simulink model "ISReferenceApplication"  (R2024b)
settings: Solver=ode4  StartTime=0.0  StopTime=60  FixedStep=1e-3  RelTol=5e-2
model workspace (MAT data in the model file):
  Downshift_Speeds = [9.5625 12.9375 16.3125 19.6875 23.0625 26.4375 29.8125 33.1875 36.5625 39.9375 43.3125 46.6875 ... (28 elements, 4x7)]
  EngRevLim = 7000
  Pedal_Positions = [0.1 0.4 0.5 0.9]
  Upshift_Speeds = [12.9375 16.3125 19.6875 33 26.4375 29.8125 33.1875 52.5 39.9375 43.3125 46.6875 77.25 ... (28 elements, 4x7)]
  VEH : object (value not decoded)
  rayDirections = [0 0 0 0 0 0 0 0 0 0 0 0 ... (363 elements, 121x3)]
  rayLengths = [20 20 20 20 20 20 20 20 20 20 20 20 ... (121 elements, 121x1)]
  rayOrigins = [0.5 0.4 0.3 0.2 0.1 0 -0.1 -0.2 -0.3 -0.4 -0.5 0.5 ... (363 elements, 121x3)]
  temp : object (value not decoded)
symbols that are objects in the model workspace (value not decoded): temp, VEH
undefined symbols (not defined in the file): DiscIntNeverNeededParam, Sim3dSensor
libraries: simulink x14, autolibutils x7, slpidlib x2, vehdynlibviscommon x2, sim3dgroundtruthsensorlib x2, autolibtranscontrolscommon x1, autolibshared x1, vehdynlibdriver x1, sharedtransform x1, vehdynlibsens x1, vehdynlibscenariocommon x1, sim3dlib x1
(part 3 of 4)

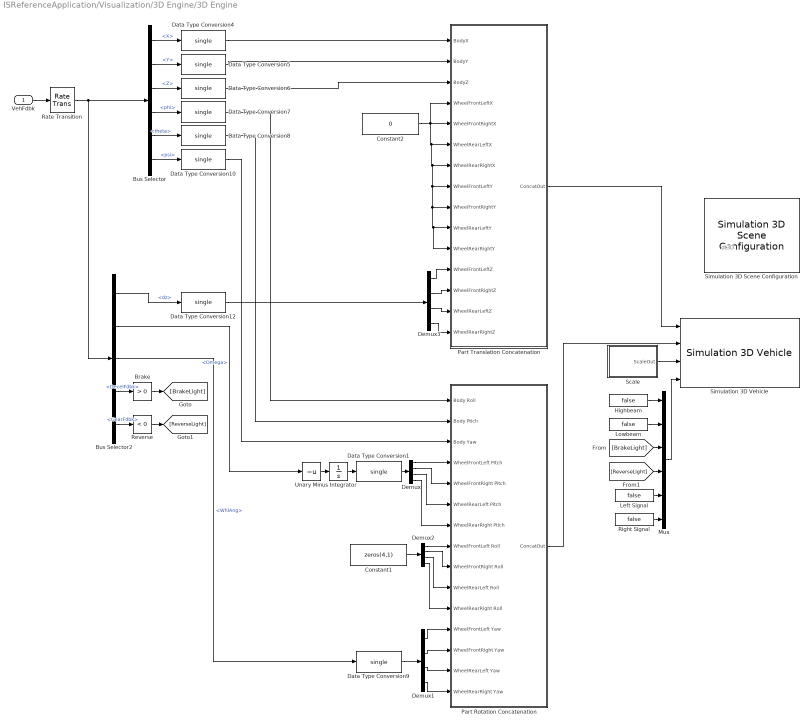
== system ISReferenceApplication/Visualization/3D Engine/3D Engine ==
  note: dt3D
  VehFdbk : Inport
  Brake : simulink/Logic and Bit Operations/Compare To Constant  relop=>  const=0  OutDataTypeStr=boolean  ZeroCross=off
  Bus Selector : BusSelector  OutputSignals=Body.InertFrm.Geom.Disp.X,Body.InertFrm.Geom.Disp.Y,Body.InertFrm.Geom.Disp.Z,Body.InertFrm.Cg.Ang.phi,Body.InertFrm.Cg.Ang.theta,Body.InertFrm.Cg.Ang.psi
  Bus Selector2 : BusSelector  OutputSignals=Wheels.TireFrame.dz,Wheels.TireFrame.Omega,Driveline.WhlAng,Driver.DecelFdbk,Driver.GearFdbk
  Constant1 : Constant  Value=zeros(4,1)  OutDataTypeStr=single
  Constant2 : Constant  Value=0  OutDataTypeStr=single
  Data Type Conversion{1,4..10,12} (9 alike) : DataTypeConversion  OutDataTypeStr=single  SaturateOnIntegerOverflow=off  RndMeth=Floor
  Demux{,1..3} (4 alike) : Demux
  Highbeam : Constant  Value=false
  Integrator : Integrator  WrapState=on  WrappedStateUpperValue=2*pi  WrappedStateLowerValue=0  ZeroCross=off
  Left Signal : Constant  Value=false
  Lowbeam : Constant  Value=false
  Mux : Mux  Inputs=6
  Part Rotation Concatenation : Subsystem
  Part Translation Concatenation : Subsystem
  Rate Transition : RateTransition  OutPortSampleTime=dt3D
  Reverse : simulink/Logic and Bit Operations/Compare To Constant  relop=<  const=0  OutDataTypeStr=boolean  ZeroCross=off
  Right Signal : Constant  Value=false
  Scale : Subsystem
  Simulation 3D Scene Configuration : sim3dlib/Simulation 3D Scene Configuration  Priority=0  ProjectFormat=Default Scenes  SceneDesc=Open surface  ProjectName=C:\Program Files\MATLAB\R2024b\toolbox\shared\sim3d_projects\automotive_project_windows\UE\WindowsNoEditor\VehicleSimulation.exe  ScenePath=/Game/Maps/HwStrght  EnableOpenDRIVE=off  vehTagList={'Custom';'Scene Origin';'SimulinkVehicle1'}  vehTag=SimulinkVehicle1  FreeCameraInitialTranslation=[0, 0, 0]  FreeCameraDefaultInitialTranslation=[-6, 0, 2]  FreeCameraInitialRotation=[0, 0, 0]  FreeCameraDefaultInitialRotation=[0, -15, 0]  OpVisEn=off  Ts=dt3D  EnableWindow=on  EnableRemoteAccess=off  EnableWeather=off  SunAzimuth=90  SunAltitude=40.0  EnableGeospatialSun=off  Latitude=0  Longitude=0  Date=2023-01-01  Time=10:30:00  GeoTimeZone=-5.0  SunDaylightSaving=off  wind=1  clouds=10  EnableVolumetricClouds=off  CloudCoverage=0  CloudAltitude=6  fog=0  rain=0  RaindropsEffect=off  SnowDensity=0  EnableGeospatial=off  UseTrueOrigin=off  OriginHeight=200  OriginLatitude=40.744652  OriginLongitude=-73.988864  MapStyle=Aerial  AdditionalAssetIDs=[]  UseAdvancedSunSky=off  SolarTime=11  TimeZone=-5  Day=21  Month=9  Year=2022  UseDaylightSavingTime=on  DSTStartDay=10  DSTStartMonth=3  DSTEndDay=3  DSTEndMonth=11  DSTSwitchHour=2  sensorTag=MainCamera1  sensorId=1  sensorName=MainCamera1  mountLoc=Origin  offsetFlag=off  tmountOffset=[0, 0, 0]  rmountOffset=[0, 0, 0]  HorizontalResolution=1280  VerticalResolution=720  HorizontalFOV=60  mountPoint=[0 0 0]  mountOrientation=[0 0 0]  aMode=2  ID=1  GeoTrigger=Inactive
      settings: LibrarySourceBlock=vdynlib/Vehicle Scenarios/Sim3D/Sim3D Core/Simulation 3D Scene Configuration
  Simulation 3D Vehicle : sim3dautolib/Simulation 3D Vehicle  Priority=-1  PassVehMesh=Sport utility vehicle  MeshPath=/MathWorksSimulation/Vehicles/Muscle/Meshes/SK_MuscleCar.SK_MuscleCar  VehColor=Red  ActorName=SimulinkVehicle1  VehLightsControl=on  HeadlightColor=[ 1, 1, 1 ]  HighBeamIntensity=100000  LowBeamIntensity=60000  HighBeamConeAngle=1.22  LowBeamConeAngle=1.22  LeftHeadlightOrientation=[ 0, 0 ]  RightHeadlightOrientation=[ 0, 0 ]  BrakelightIntensity=500  ReverselightIntensity=500  SignallightIntensity=500  SignallightPeriod=1  SignalPulseWidth=50  Translation=[VEH.InitialLongPosition VEH.InitialLatPosition -VEH.InitialVertPosition; 0 0 0; 0 0 0; 0 0 0; 0 0 0]  Rotation=[VEH.InitialRollAngle VEH.InitialPitchAngle VEH.InitialYawAngle; 0 0 0; 0 0 0; 0 0 0; 0 0 0]  Scale=ones( 5, 3 )  SampleTime=dt3D  ActorType=SimulinkVehicle  ID=1  aMode=2  ActorTag=SimulinkVehicle1
  Unary Minus : UnaryMinus
  wires:
  Unary Minus/1 -> Integrator/1
  Bus Selector2/1 -> Data Type Conversion12/1  "<dz>"
  Rate Transition/1 -> Bus Selector/1, Bus Selector2/1
  Scale/1(ScaleOut) -> Simulation 3D Vehicle/3
  Demux/4 -> Part Rotation Concatenation/7(WheelRearRight Ptich)
  Demux/3 -> Part Rotation Concatenation/6(WheelRearLeft Pitch)
  Demux/2 -> Part Rotation Concatenation/5(WheelFrontRight Pitch)
  Demux/1 -> Part Rotation Concatenation/4(WheelFrontLeft Pitch)
  Constant1/1 -> Demux2/1
  Bus Selector/4 -> Data Type Conversion7/1  "<phi>"
  Part Rotation Concatenation/1(ConcatOut) -> Simulation 3D Vehicle/2
  Part Translation Concatenation/1(ConcatOut) -> Simulation 3D Vehicle/1
  Data Type Conversion12/1 -> Demux3/1
  Demux3/4 -> Part Translation Concatenation/15(WheelRearRightZ)
  Demux3/3 -> Part Translation Concatenation/14(WheelRearLeftZ)
  Demux3/1 -> Part Translation Concatenation/12(WheelFrontLeftZ)
  Demux3/2 -> Part Translation Concatenation/13(WheelFrontRightZ)
  VehFdbk/1 -> Rate Transition/1
  Data Type Conversion6/1 -> Part Translation Concatenation/3(BodyZ)
  Demux1/4 -> Part Rotation Concatenation/15(WheelRearRight Yaw)
  Demux1/3 -> Part Rotation Concatenation/14(WheelRearLeft Yaw)
  Demux2/1 -> Part Rotation Concatenation/8(WheelFrontLeft Roll)
  Demux2/2 -> Part Rotation Concatenation/9(WheelFrontRight Roll)
  Demux2/3 -> Part Rotation Concatenation/10(WheelRearLeft Roll)
  Demux2/4 -> Part Rotation Concatenation/11(WheelRearRight Roll)
  Bus Selector2/3 -> Data Type Conversion9/1  "<WhlAng>"
  Bus Selector2/2 -> Unary Minus/1  "<Omega>"
  Data Type Conversion9/1 -> Demux1/1
  Demux1/1 -> Part Rotation Concatenation/12(WheelFrontLeft Yaw)
  Demux1/2 -> Part Rotation Concatenation/13(WheelFrontRight Yaw)
  Integrator/1 -> Data Type Conversion1/1
  Data Type Conversion1/1 -> Demux/1
  Data Type Conversion8/1 -> Part Rotation Concatenation/2(Body Ptich)
  Data Type Conversion5/1 -> Part Translation Concatenation/2(BodyY)
  Data Type Conversion10/1 -> Part Rotation Concatenation/3(Body Yaw)
  Constant2/1 -> Part Translation Concatenation/5(WheelFrontRightX), Part Translation Concatenation/6(WheelRearLeftX), Part Translation Concatenation/7(WheelRearRightX), Part Translation Concatenation/8(WheelFrontLeftY), Part Translation Concatenation/9(WheelFrontRightY), Part Translation Concatenation/10(WheelRearLeftY), Part Translation Concatenation/11(WheelRearRightY), Part Translation Concatenation/4(WheelFrontLeftX)
  Data Type Conversion4/1 -> Part Translation Concatenation/1(BodyX)
  Data Type Conversion7/1 -> Part Rotation Concatenation/1(Body Roll)
  Bus Selector/1 -> Data Type Conversion4/1  "<X>"
  Bus Selector/2 -> Data Type Conversion5/1  "<Y>"
  Bus Selector/3 -> Data Type Conversion6/1  "<Z>"
  Bus Selector/6 -> Data Type Conversion10/1  "<psi>"
  Bus Selector/5 -> Data Type Conversion8/1  "<theta>"
  [BrakeLight] -> Mux/3
  Mux/1 -> Simulation 3D Vehicle/4
  Brake/1 -> [BrakeLight]
  Highbeam/1 -> Mux/1
  Reverse/1 -> [ReverseLight]
  [ReverseLight] -> Mux/4
  Lowbeam/1 -> Mux/2
  Right Signal/1 -> Mux/6
  Left Signal/1 -> Mux/5
  Bus Selector2/4 -> Brake/1  "<DecelFdbk>"
  Bus Selector2/5 -> Reverse/1  "<GearFdbk>"

== system ISReferenceApplication/Visualization/3D Engine/3D Engine Disabled ==
  VehFdbk : Inport
  Terminator : Terminator
  wires:
  VehFdbk/1 -> Terminator/1

== system ISReferenceApplication/Visualization/ISO 15037-1:2006/Disabled ==
  VehFdbk : Inport
  Terminator1 : Terminator
  wires:
  VehFdbk/1 -> Terminator1/1

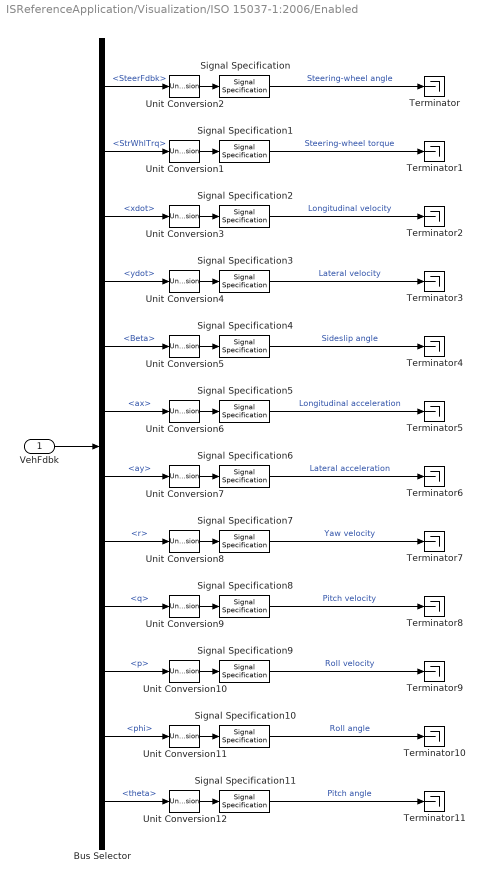
== system ISReferenceApplication/Visualization/ISO 15037-1:2006/Enabled ==
  VehFdbk : Inport
  Bus Selector : BusSelector  OutputSignals=Driver.SteerFdbk,Steering.StrWhlTrq,Body.BdyFrm.Cg.Vel.xdot,Body.BdyFrm.Cg.Vel.ydot,Body.BdyFrm.Cg.Ang.Beta,Body.BdyFrm.Cg.Acc.ax,Body.BdyFrm.Cg.Acc.ay,Body.BdyFrm.Cg.AngVel.r,Body.BdyFrm.Cg.AngVel.q,Body.BdyFrm.Cg.AngVel.p,Body.InertFrm.Cg.Ang.phi,Body.InertFrm.Cg.Ang.theta
  Signal Specification{,4,10..11} (4 alike) : SignalSpecification  Unit=deg
  Signal Specification1 : SignalSpecification  Unit=N*m
  Signal Specification2 : SignalSpecification  Unit=km/h
  Signal Specification3 : SignalSpecification  Unit=m/s
  Signal Specification5 : SignalSpecification  Unit=m/s^2
  Signal Specification6 : SignalSpecification  Unit=m/s^2
  Signal Specification7 : SignalSpecification  Unit=deg/s
  Signal Specification8 : SignalSpecification  Unit=deg/s
  Signal Specification9 : SignalSpecification  Unit=deg/s
  Terminator{,1..11} (12 alike) : Terminator
  Unit Conversion{1..12} (12 alike) : UnitConversion
  wires:
  Bus Selector/12 -> Unit Conversion12/1  "<theta>"
  Signal Specification11/1 -> Terminator11/1  "Pitch angle"
  Unit Conversion12/1 -> Signal Specification11/1
  Bus Selector/11 -> Unit Conversion11/1  "<phi>"
  Unit Conversion11/1 -> Signal Specification10/1
  Signal Specification10/1 -> Terminator10/1  "Roll angle"
  Bus Selector/10 -> Unit Conversion10/1  "<p>"
  Signal Specification9/1 -> Terminator9/1  "Roll velocity"
  Unit Conversion10/1 -> Signal Specification9/1
  Bus Selector/9 -> Unit Conversion9/1  "<q>"
  Unit Conversion9/1 -> Signal Specification8/1
  Signal Specification8/1 -> Terminator8/1  "Pitch velocity"
  Bus Selector/8 -> Unit Conversion8/1  "<r>"
  Signal Specification7/1 -> Terminator7/1  "Yaw velocity"
  Unit Conversion8/1 -> Signal Specification7/1
  Bus Selector/7 -> Unit Conversion7/1  "<ay>"
  Unit Conversion7/1 -> Signal Specification6/1
  Signal Specification6/1 -> Terminator6/1  "Lateral acceleration"
  Bus Selector/6 -> Unit Conversion6/1  "<ax>"
  Signal Specification5/1 -> Terminator5/1  "Longitudinal acceleration"
  Unit Conversion6/1 -> Signal Specification5/1
  Bus Selector/5 -> Unit Conversion5/1  "<Beta>"
  Unit Conversion5/1 -> Signal Specification4/1
  Signal Specification4/1 -> Terminator4/1  "Sideslip angle"
  Bus Selector/4 -> Unit Conversion4/1  "<ydot>"
  Signal Specification3/1 -> Terminator3/1  "Lateral velocity"
  Unit Conversion4/1 -> Signal Specification3/1
  Bus Selector/3 -> Unit Conversion3/1  "<xdot>"
  Unit Conversion3/1 -> Signal Specification2/1
  Signal Specification2/1 -> Terminator2/1  "Longitudinal velocity"
  Signal Specification1/1 -> Terminator1/1  "Steering-wheel torque"
  Unit Conversion1/1 -> Signal Specification1/1
  Bus Selector/2 -> Unit Conversion1/1  "<StrWhlTrq>"
  Signal Specification/1 -> Terminator/1  "Steering-wheel angle"
  Unit Conversion2/1 -> Signal Specification/1
  VehFdbk/1 -> Bus Selector/1
  Bus Selector/1 -> Unit Conversion2/1  "<SteerFdbk>"

== system ISReferenceApplication/Controllers/Brake Pressure Control/Bang Bang ABS/Bang-bang controller ==
  in_1 : Inport
  Constant : Constant  Value=0
  Data Type Conversion1 : DataTypeConversion  OutDataTypeStr=double
  Data Type Conversion2 : DataTypeConversion  OutDataTypeStr=double
  Relational Operator : RelationalOperator  Operator=>  OutDataTypeStr=boolean
  Relational Operator1 : RelationalOperator  Operator=<  OutDataTypeStr=boolean
  Sum : Sum  Inputs=+-  InputSameDT=on  SaturateOnIntegerOverflow=on  OutDataTypeStr=Inherit: Same as first input
  out_1 : Outport  InitialOutput=0  VectorParamsAs1DForOutWhenUnconnected=off
  wires:
  Data Type Conversion2/1 -> Sum/2
  Data Type Conversion1/1 -> Sum/1
  Sum/1 -> out_1/1
  Relational Operator/1 -> Data Type Conversion1/1
  Relational Operator1/1 -> Data Type Conversion2/1
  Constant/1 -> Relational Operator/2, Relational Operator1/2
  in_1/1 -> Relational Operator1/1, Relational Operator/1

== system ISReferenceApplication/Controllers/Brake Pressure Control/Bang Bang ABS/Kappa ==
  xdot : Inport
  Omega : Inport  Port=2  Partition=on  PartitionDimension=1  PartitionWidth=1  PartitionOffset=0
  For Each : ForEach  DisableCoverage=on
  MATLAB Function : MATLAB Function  TreatAsAtomicUnit=on
  KappaEst : Outport  ConcatenationDimension=1
  wires:
  MATLAB Function/1(KappaEst) -> KappaEst/1
  xdot/1 -> MATLAB Function/2(xdot)
  Omega/1 -> MATLAB Function/1(Omega)

== system ISReferenceApplication/Controllers/Brake Pressure Control/Five-State ABS and TCS/ABSCtrlForEach ==
  Pref : Inport
  WhlAccel : Inport  Port=2
  WhlSlip : Inport  Port=3
  VehSpd : Inport  Port=4
  Constant7 : Constant  Value=WhlAccelOpt
  Constant8 : Constant  Value=KappaOpt
  For Each Subsystem : Subsystem  TreatAsAtomicUnit=on
  Gain : Gain  Gain=Re
  Saturation1 : Saturate  UpperLimit=1  LowerLimit=-1
  Selector : Selector  InputPortWidth=1  IndexOptions=Index vector (dialog)  Indices=[1 1 1 1]  OutputSizes=1
  Sum : Sum  Inputs=|+-
  Sum1 : Sum  Inputs=|+-
  BrkCtrl : Outport
  BrkFlag : Outport  Port=2
  wires:
  Gain/1 -> Sum/1
  Constant8/1 -> Sum1/2
  WhlSlip/1 -> Saturation1/1
  Constant7/1 -> Sum/2
  Sum1/1 -> For Each Subsystem/1(e1)
  WhlAccel/1 -> Gain/1
  Saturation1/1 -> Sum1/1
  For Each Subsystem/2(Flag) -> BrkFlag/1
  Pref/1 -> Selector/1
  VehSpd/1 -> For Each Subsystem/4(VehSpd)
  For Each Subsystem/1(Pb) -> BrkCtrl/1  "BrkPrsCmdCtrl"
  Selector/1 -> For Each Subsystem/3(Pref)
  Sum/1 -> For Each Subsystem/2(e2)

== system ISReferenceApplication/Controllers/Brake Pressure Control/Five-State ABS and TCS/TCSCtrlForEach ==
  WhlAccel : Inport
  WhlSlip : Inport  Port=2
  AccelFdbk : Inport  Port=3
  PbFdbk : Inport  Port=4
  Constant7 : Constant  Value=WhlAccelOpt
  Constant8 : Constant  Value=KappaOpt
  For Each Subsystem : Subsystem  TreatAsAtomicUnit=on
  Gain : Gain  Gain=Re
  Interpreted MATLAB Function : MATLABFcn  MATLABFcn=abs((u(1)+u(2)) - (u(3) + u(4)))/2
  Saturation1 : Saturate  UpperLimit=1  LowerLimit=-1
  Selector : Selector  InputPortWidth=1  IndexOptions=Index vector (dialog)  Indices=[1 1 1 1]  OutputSizes=1
  Sum : Sum  Inputs=|+-
  Sum1 : Sum  Inputs=|+-
  BrkCtrl : Outport
  BrkFlag : Outport  Port=2
  wires:
  Gain/1 -> Sum/1
  Constant8/1 -> Sum1/2
  WhlSlip/1 -> Saturation1/1
  Constant7/1 -> Sum/2
  Sum1/1 -> For Each Subsystem/1(e1)
  WhlAccel/1 -> Gain/1
  Saturation1/1 -> Interpreted MATLAB Function/1, Sum1/1
  For Each Subsystem/2(Flag) -> BrkFlag/1
  AccelFdbk/1 -> Selector/1
  For Each Subsystem/1(Pb) -> BrkCtrl/1  "BrkPrsCmdCtrl"
  Selector/1 -> For Each Subsystem/4(AccelFdbk)
  Sum/1 -> For Each Subsystem/3(e2)
  Interpreted MATLAB Function/1 -> For Each Subsystem/2(Enb)
  PbFdbk/1 -> For Each Subsystem/5(PbFdbk)

== system ISReferenceApplication/Controllers/Brake Pressure Control/Five-State ABS and TCS/Wheel Accel and Slip Estimator ==
  Omega : Inport
  Accel : Inport  Port=2
  Demux : Demux  Outputs=3
  Discrete-Time Integrator : DiscreteIntegrator  IntegratorMethod=Integration: Trapezoidal  SampleTime=-1  ICPrevOutput=DiscIntNeverNeededParam  ICPrevScaledInput=DiscIntNeverNeededParam
  Kappa : Subsystem  TreatAsAtomicUnit=on
  Terminator : Terminator
  Terminator1 : Terminator
  Wheel Accel : Subsystem  TreatAsAtomicUnit=on
  <WhlAccel> : Outport
  <Kappa> : Outport  Port=2
  <xdot> : Outport  Port=3
  wires:
  Accel/1 -> Demux/1
  Discrete-Time Integrator/1 -> <xdot>/1, Kappa/1(xdot)
  Demux/1 -> Discrete-Time Integrator/1
  Demux/2 -> Terminator/1
  Demux/3 -> Terminator1/1
  Omega/1 -> Kappa/2(Omega), Wheel Accel/1(Omega)
  Wheel Accel/1(WhlAccel) -> <WhlAccel>/1
  Kappa/1(KappaEst) -> <Kappa>/1

== system ISReferenceApplication/Controllers/ECU/Torque Cmd/Rev Limiter Control ==
  TrqCmd : Inport
  EngSpd : Inport  Port=2
  1-D Lookup Table : Lookup_n-D  NumberOfTableDimensions=1  BreakpointsForDimension1=[1 1.01]  Table=[1 0]  ExtrapMethod=Clip  InternalRulePriority=Speed  RndMeth=Simplest
  Constant : Constant  Value=EngRevLim
  Product : Product
  Product1 : Product  Inputs=*/
  TrqCmdRevLimited : Outport  VectorParamsAs1DForOutWhenUnconnected=off
  wires:
  EngSpd/1 -> Product1/1
  Product/1 -> TrqCmdRevLimited/1
  1-D Lookup Table/1 -> Product/2
  TrqCmd/1 -> Product/1
  Constant/1 -> Product1/2
  Product1/1 -> 1-D Lookup Table/1

== system ISReferenceApplication/Controllers/Transmission Controller/Transmission Controller/TCM ==
  AccCmd : Inport
  EngSpd : Inport  Port=2
  Omega : Inport  Port=3  Unit=rad/s
  function : TriggerPort  TriggerType=function-call  VariantControl=Variant
  Gain : Gain  Gain=.3065/4
  Neutral Select : Subsystem
  Signal Specification1 : SignalSpecification  Unit=m/s
  Signal Specification2 : SignalSpecification  Unit=km/hr
  Speed LPF : DiscreteTransferFcn  Numerator=[0.000000000000000 0.009950166250832 ]  Denominator=[1.000000000000000 -0.990049833749168 ]  mask(DiscretizedDiscreteTransferFcn){}
      mask init:
      | %zoh
  Sum of Elements : Sum  Inputs=+
  TCM Shift Controller : Stateflow chart  TreatAsAtomicUnit=on
  Unit Conversion1 : UnitConversion
  GearCmd : Outport  VectorParamsAs1DForOutWhenUnconnected=off
  wires:
  Signal Specification2/1 -> Speed LPF/1
  TCM Shift Controller/1(GearCmd) -> GearCmd/1  "GearCmd"
  AccCmd/1 -> Neutral Select/1(AccCmd), TCM Shift Controller/2(pedal)  "AccCmd"
  Neutral Select/1(Neutral Select) -> TCM Shift Controller/3(Neutral)
  EngSpd/1 -> Neutral Select/2(EngSpd)
  Speed LPF/1 -> TCM Shift Controller/1(speed)
  Unit Conversion1/1 -> Signal Specification2/1
  Omega/1 -> Sum of Elements/1
  Gain/1 -> Signal Specification1/1
  Signal Specification1/1 -> Unit Conversion1/1
  Sum of Elements/1 -> Gain/1

== system ISReferenceApplication/Environment/Ground Feedback/3D Engine/3D Engine Source ==
  VehFdbk : Inport
  Multiple Points : Subsystem  VariantControl=terrType==2
  Single Point : Subsystem  VariantControl=terrType ==1
  z : Outport
  DCM : Outport  Port=2

== system ISReferenceApplication/Visualization/3D Engine/3D Engine/Part Rotation Concatenation ==
  Body Roll : Inport
  Body Ptich : Inport  Port=2
  Body Yaw : Inport  Port=3
  WheelFrontLeft Pitch : Inport  Port=4
  WheelFrontRight Pitch : Inport  Port=5
  WheelRearLeft Pitch : Inport  Port=6
  WheelRearRight Ptich : Inport  Port=7
  WheelFrontLeft Roll : Inport  Port=8
  WheelFrontRight Roll : Inport  Port=9
  WheelRearLeft Roll : Inport  Port=10
  WheelRearRight Roll : Inport  Port=11
  WheelFrontLeft Yaw : Inport  Port=12
  WheelFrontRight Yaw : Inport  Port=13
  WheelRearLeft Yaw : Inport  Port=14
  WheelRearRight Yaw : Inport  Port=15
  AllParts : Concatenate  NumInputs=5  Mode=Multidimensional array
  Body : Concatenate  NumInputs=3  Mode=Multidimensional array  ConcatenateDimension=2
  WheelFrontLeft : Concatenate  NumInputs=3  Mode=Multidimensional array  ConcatenateDimension=2
  WheelFrontRight : Concatenate  NumInputs=3  Mode=Multidimensional array  ConcatenateDimension=2
  WheelRearLeft : Concatenate  NumInputs=3  Mode=Multidimensional array  ConcatenateDimension=2
  WheelRearRight : Concatenate  NumInputs=3  Mode=Multidimensional array  ConcatenateDimension=2
  ConcatOut : Outport  VectorParamsAs1DForOutWhenUnconnected=off
  wires:
  Body Yaw/1 -> Body/3
  WheelFrontLeft Yaw/1 -> WheelFrontLeft/3
  WheelFrontLeft/1 -> AllParts/2
  Body/1 -> AllParts/1
  WheelRearLeft/1 -> AllParts/4
  WheelFrontRight/1 -> AllParts/3
  WheelRearRight Yaw/1 -> WheelRearRight/3
  WheelRearLeft Yaw/1 -> WheelRearLeft/3
  AllParts/1 -> ConcatOut/1
  WheelRearRight/1 -> AllParts/5
  WheelFrontRight Yaw/1 -> WheelFrontRight/3
  Body Roll/1 -> Body/1
  Body Ptich/1 -> Body/2
  WheelFrontLeft Pitch/1 -> WheelFrontLeft/2
  WheelFrontLeft Roll/1 -> WheelFrontLeft/1
  WheelFrontRight Roll/1 -> WheelFrontRight/1
  WheelFrontRight Pitch/1 -> WheelFrontRight/2
  WheelRearLeft Roll/1 -> WheelRearLeft/1
  WheelRearLeft Pitch/1 -> WheelRearLeft/2
  WheelRearRight Roll/1 -> WheelRearRight/1
  WheelRearRight Ptich/1 -> WheelRearRight/2

== system ISReferenceApplication/Visualization/3D Engine/3D Engine/Part Translation Concatenation ==
  BodyX : Inport
  BodyY : Inport  Port=2
  BodyZ : Inport  Port=3
  WheelFrontLeftX : Inport  Port=4
  WheelFrontRightX : Inport  Port=5
  WheelRearLeftX : Inport  Port=6
  WheelRearRightX : Inport  Port=7
  WheelFrontLeftY : Inport  Port=8
  WheelFrontRightY : Inport  Port=9
  WheelRearLeftY : Inport  Port=10
  WheelRearRightY : Inport  Port=11
  WheelFrontLeftZ : Inport  Port=12
  WheelFrontRightZ : Inport  Port=13
  WheelRearLeftZ : Inport  Port=14
  WheelRearRightZ : Inport  Port=15
  AllParts : Concatenate  NumInputs=5  Mode=Multidimensional array
  Body : Concatenate  NumInputs=3  Mode=Multidimensional array  ConcatenateDimension=2
  WheelFrontLeft : Concatenate  NumInputs=3  Mode=Multidimensional array  ConcatenateDimension=2
  WheelFrontRight : Concatenate  NumInputs=3  Mode=Multidimensional array  ConcatenateDimension=2
  WheelRearLeft : Concatenate  NumInputs=3  Mode=Multidimensional array  ConcatenateDimension=2
  WheelRearRight : Concatenate  NumInputs=3  Mode=Multidimensional array  ConcatenateDimension=2
  ConcatOut : Outport  VectorParamsAs1DForOutWhenUnconnected=off
  wires:
  BodyX/1 -> Body/1
  BodyZ/1 -> Body/3
  WheelFrontLeftX/1 -> WheelFrontLeft/1
  WheelFrontLeftZ/1 -> WheelFrontLeft/3
  WheelFrontLeftY/1 -> WheelFrontLeft/2
  BodyY/1 -> Body/2
  WheelFrontLeft/1 -> AllParts/2
  WheelRearRightX/1 -> WheelRearRight/1
  Body/1 -> AllParts/1
  WheelRearLeft/1 -> AllParts/4
  WheelFrontRight/1 -> AllParts/3
  WheelRearRightZ/1 -> WheelRearRight/3
  WheelFrontRightY/1 -> WheelFrontRight/2
  WheelFrontRightX/1 -> WheelFrontRight/1
  WheelRearRightY/1 -> WheelRearRight/2
  WheelRearLeftZ/1 -> WheelRearLeft/3
  AllParts/1 -> ConcatOut/1
  WheelRearLeftY/1 -> WheelRearLeft/2
  WheelRearRight/1 -> AllParts/5
  WheelRearLeftX/1 -> WheelRearLeft/1
  WheelFrontRightZ/1 -> WheelFrontRight/3

== system ISReferenceApplication/Visualization/3D Engine/3D Engine/Scale ==
  Constant{1..12,17,32..33} (15 alike) : Constant  OutDataTypeStr=single
  PartConcatenation : Subsystem
  ScaleOut : Outport  VectorParamsAs1DForOutWhenUnconnected=off
  wires:
  Constant10/1 -> PartConcatenation/15(WheelRearRightZ)
  Constant9/1 -> PartConcatenation/14(WheelRearRightY)
  Constant11/1 -> PartConcatenation/13(WheelRearRightX)
  Constant7/1 -> PartConcatenation/12(WheelRearLeftZ)
  Constant6/1 -> PartConcatenation/11(WheelRearLeftY)
  Constant8/1 -> PartConcatenation/10(WheelRearLeftX)
  Constant4/1 -> PartConcatenation/9(WheelFrontRightZ)
  Constant3/1 -> PartConcatenation/8(WheelFrontRightY)
  Constant5/1 -> PartConcatenation/7(WheelFrontRightX)
  Constant2/1 -> PartConcatenation/6(WheelFrontLeftZ)
  Constant1/1 -> PartConcatenation/5(WheelFrontLeftY)
  Constant33/1 -> PartConcatenation/4(WheelFrontLeftX)
  Constant32/1 -> PartConcatenation/3(BodyZ)
  Constant17/1 -> PartConcatenation/2(BodyY)
  Constant12/1 -> PartConcatenation/1(BodyX)
  PartConcatenation/1(ConcatOut) -> ScaleOut/1

== system ISReferenceApplication/Controllers/Brake Pressure Control/Five-State ABS and TCS/ABSCtrlForEach/For Each Subsystem ==
  e1 : Inport  Partition=on  PartitionDimension=1  PartitionWidth=1  PartitionOffset=0
  e2 : Inport  Port=2  Partition=on  PartitionDimension=1  PartitionWidth=1  PartitionOffset=0
  Pref : Inport  Port=3  Partition=on  PartitionDimension=1  PartitionWidth=1  PartitionOffset=0
  VehSpd : Inport  Port=4
  ABSForEachWheel : Stateflow chart  InitFcn=[~]=vehdynicon('vehdynblk',gcb);  TreatAsAtomicUnit=on
  For Each : ForEach  DisableCoverage=on
  Saturation2 : Saturate  UpperLimit=1  LowerLimit=0  ZeroCross=off
  Pb : Outport  ConcatenationDimension=1
  Flag : Outport  Port=2  ConcatenationDimension=1
  wires:
  e1/1 -> ABSForEachWheel/1(e1)
  e2/1 -> ABSForEachWheel/2(e2)
  VehSpd/1 -> ABSForEachWheel/4(VehSpd)
  Saturation2/1 -> Pb/1  "BrkPrsCmdCtrl"
  ABSForEachWheel/2(Flag) -> Flag/1
  ABSForEachWheel/1(PbOutput) -> Saturation2/1
  Pref/1 -> ABSForEachWheel/3(Pref)

== system ISReferenceApplication/Controllers/Brake Pressure Control/Five-State ABS and TCS/TCSCtrlForEach/For Each Subsystem ==
  e1 : Inport  Partition=on  PartitionDimension=1  PartitionWidth=1  PartitionOffset=0
  Enb : Inport  Port=2
  e2 : Inport  Port=3  Partition=on  PartitionDimension=1  PartitionWidth=1  PartitionOffset=0
  AccelFdbk : Inport  Port=4  Partition=on  PartitionDimension=1  PartitionWidth=1  PartitionOffset=0
  PbFdbk : Inport  Port=5  Partition=on  PartitionDimension=1  PartitionWidth=1  PartitionOffset=0
  ABSForEachWheel : Stateflow chart  InitFcn=[~]=vehdynicon('vehdynblk',gcb);  TreatAsAtomicUnit=on
  Discrete-Time Integrator1 : DiscreteIntegrator  IntegratorMethod=Integration: Trapezoidal  ExternalReset=rising  SampleTime=-1  LimitOutput=on  UpperSaturationLimit=1  LowerSaturationLimit=0  ICPrevOutput=DiscIntNeverNeededParam  ICPrevScaledInput=DiscIntNeverNeededParam
  For Each : ForEach  DisableCoverage=on
  IsNegative : simulink/Logic and Bit Operations/Compare To Zero  relop===  OutDataTypeStr=boolean  ZeroCross=off
  Pb : Outport  ConcatenationDimension=1
  Flag : Outport  Port=2  ConcatenationDimension=1
  wires:
  e1/1 -> ABSForEachWheel/1(e1)
  e2/1 -> ABSForEachWheel/2(e2)
  Discrete-Time Integrator1/1 -> Pb/1  "BrkPrsCmdCtrl"
  ABSForEachWheel/2(Flag) -> IsNegative/1, Flag/1
  ABSForEachWheel/1(PbOutput) -> Discrete-Time Integrator1/1
  AccelFdbk/1 -> ABSForEachWheel/3(AccelFdbk)
  Enb/1 -> ABSForEachWheel/4(Enb)
  PbFdbk/1 -> ABSForEachWheel/5(Pb)
  IsNegative/1 -> Discrete-Time Integrator1/2

== system ISReferenceApplication/Controllers/Brake Pressure Control/Five-State ABS and TCS/Wheel Accel and Slip Estimator/Kappa ==
  xdot : Inport
  Omega : Inport  Port=2  PortDimensions=1  Partition=on  PartitionDimension=1  PartitionWidth=1  PartitionOffset=0
  For Each : ForEach  DisableCoverage=on
  MATLAB Function : MATLAB Function  TreatAsAtomicUnit=on
  KappaEst : Outport  ConcatenationDimension=1
  wires:
  MATLAB Function/1(KappaEst) -> KappaEst/1
  xdot/1 -> MATLAB Function/2(xdot)
  Omega/1 -> MATLAB Function/1(Omega)

== system ISReferenceApplication/Controllers/Brake Pressure Control/Five-State ABS and TCS/Wheel Accel and Slip Estimator/Wheel Accel ==
  Omega : Inport  PortDimensions=1  Partition=on  PartitionDimension=1  PartitionWidth=1  PartitionOffset=0
  For Each : ForEach  DisableCoverage=on
  SG Diff : autolibutils/SG Diff  N=2  F=500  div0Tol=.001  aMode=2
  Terminator : Terminator
  WhlAccel : Outport  ConcatenationDimension=1
  wires:
  Omega/1 -> SG Diff/1
  SG Diff/1 -> Terminator/1
  SG Diff/2 -> WhlAccel/1

== system ISReferenceApplication/Controllers/Transmission Controller/Transmission Controller/TCM/Neutral Select ==
  AccCmd : Inport
  EngSpd : Inport  Port=2
  Constant : Constant  Value=1200
  Constant1 : Constant  Value=1e-2
  Constant2 : Constant  Value=500
  Logical Operator : Logic  AllPortsSameDT=off  OutDataTypeStr=boolean
  Logical Operator1 : Logic  Operator=OR  AllPortsSameDT=off  OutDataTypeStr=boolean
  Relational Operator : RelationalOperator  Operator=<=  OutDataTypeStr=boolean  ZeroCross=off  RndMeth=Simplest  InputSameDT=off
  Relational Operator1 : RelationalOperator  Operator=<=  OutDataTypeStr=boolean  ZeroCross=off  RndMeth=Simplest  InputSameDT=off
  Relational Operator2 : RelationalOperator  Operator=<=  OutDataTypeStr=boolean  ZeroCross=off  RndMeth=Simplest  InputSameDT=off
  Neutral Select : Outport  VectorParamsAs1DForOutWhenUnconnected=off
  wires:
  EngSpd/1 -> Relational Operator/1, Relational Operator2/1
  Relational Operator1/1 -> Logical Operator/1
  AccCmd/1 -> Relational Operator1/1
  Constant1/1 -> Relational Operator1/2
  Logical Operator1/1 -> Neutral Select/1
  Constant/1 -> Relational Operator/2
  Relational Operator/1 -> Logical Operator/2
  Logical Operator/1 -> Logical Operator1/1
  Constant2/1 -> Relational Operator2/2
  Relational Operator2/1 -> Logical Operator1/2

== system ISReferenceApplication/Controllers/Transmission Controller/Transmission Controller/TCM/TCM Shift Controller/calc ==
  note: Determine if next gear will be
      | higher or lower than current gear
  gear : Inport  OutDataTypeStr=double  PortDimensions=1
  pedal : Inport  Port=2  OutDataTypeStr=double  PortDimensions=1
  speed : Inport  Port=3  OutDataTypeStr=double  PortDimensions=1
  f : TriggerPort  TriggerType=function-call  VariantControl=Variant  StatesWhenEnabling=reset
      settings: CopyFcn=Stateflow.SLINSF.SimulinkMan.removeBlockPreDeleteFcn  PreDeleteFcn=Stateflow.SLINSF.SimulinkMan.unsafePredeleteFcn
  Add1 : Sum  Inputs=+-
  Add3 : Sum  Inputs=+-
  Add4 : Sum  Inputs=+-
  Calculate Upshift Threshold : Lookup_n-D  BreakpointsForDimension1=Pedal_Positions  BreakpointsForDimension2=1:7  Table=Upshift_Speeds  ExtrapMethod=Clip  UseLastTableValue=on  InternalRulePriority=Speed  RndMeth=Simplest
      settings: InputPortMap=u0,u1
  Calculate Downshift Threshold : Lookup_n-D  BreakpointsForDimension1=Pedal_Positions  BreakpointsForDimension2=2:8  Table=Downshift_Speeds  ExtrapMethod=Clip  UseLastTableValue=on  InternalRulePriority=Speed  RndMeth=Simplest
      settings: InputPortMap=u0,u1
  SpdThr : Outport  VectorParamsAs1DForOutWhenUnconnected=off
  wires:
  pedal/1 -> Calculate Downshift Threshold/1, Calculate Upshift Threshold/1
  gear/1 -> Calculate Downshift Threshold/2, Calculate Upshift Threshold/2
  Calculate Downshift Threshold/1 -> Add3/2
  Calculate Upshift Threshold/1 -> Add1/1
  speed/1 -> Add1/2, Add3/1
  Add1/1 -> Add4/1
  Add3/1 -> Add4/2
  Add4/1 -> SpdThr/1

== system ISReferenceApplication/Controllers/Transmission Controller/Transmission Controller/TCM/TCM Shift Controller/calc_down ==
  gear : Inport  OutDataTypeStr=double  PortDimensions=1
  pedal : Inport  Port=2  OutDataTypeStr=double  PortDimensions=1
  f : TriggerPort  TriggerType=function-call  VariantControl=Variant  StatesWhenEnabling=reset
      settings: CopyFcn=Stateflow.SLINSF.SimulinkMan.removeBlockPreDeleteFcn  PreDeleteFcn=Stateflow.SLINSF.SimulinkMan.unsafePredeleteFcn
  Calculate Downshift Threshold : Lookup_n-D  BreakpointsForDimension1=Pedal_Positions  BreakpointsForDimension2=2:8  Table=Downshift_Speeds  ExtrapMethod=Clip  UseLastTableValue=on  InternalRulePriority=Speed  RndMeth=Simplest
      settings: InputPortMap=u0,u1
  down_th : Outport  VectorParamsAs1DForOutWhenUnconnected=off
  wires:
  Calculate Downshift Threshold/1 -> down_th/1
  gear/1 -> Calculate Downshift Threshold/2
  pedal/1 -> Calculate Downshift Threshold/1

== system ISReferenceApplication/Controllers/Transmission Controller/Transmission Controller/TCM/TCM Shift Controller/calc_up ==
  gear : Inport  OutDataTypeStr=double  PortDimensions=1
  pedal : Inport  Port=2  OutDataTypeStr=double  PortDimensions=1
  f : TriggerPort  TriggerType=function-call  VariantControl=Variant  StatesWhenEnabling=reset
      settings: CopyFcn=Stateflow.SLINSF.SimulinkMan.removeBlockPreDeleteFcn  PreDeleteFcn=Stateflow.SLINSF.SimulinkMan.unsafePredeleteFcn
  Calculate Upshift Threshold : Lookup_n-D  BreakpointsForDimension1=Pedal_Positions  BreakpointsForDimension2=1:7  Table=Upshift_Speeds  ExtrapMethod=Clip  UseLastTableValue=on  InternalRulePriority=Speed  RndMeth=Simplest
      settings: InputPortMap=u0,u1
  up_th : Outport  VectorParamsAs1DForOutWhenUnconnected=off
  wires:
  Calculate Upshift Threshold/1 -> up_th/1
  pedal/1 -> Calculate Upshift Threshold/1
  gear/1 -> Calculate Upshift Threshold/2

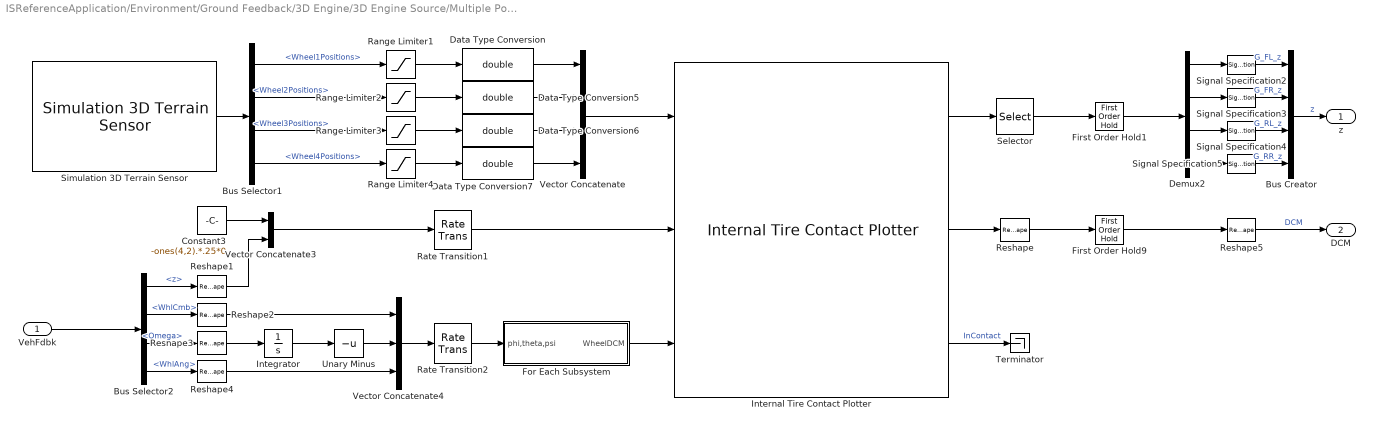
== system ISReferenceApplication/Environment/Ground Feedback/3D Engine/3D Engine Source/Multiple Points ==
  VehFdbk : Inport
  Bus Creator : BusCreator  Inputs=4
  Bus Selector1 : BusSelector  OutputSignals=Wheel1Positions,Wheel2Positions,Wheel3Positions,Wheel4Positions
  Bus Selector2 : BusSelector  OutputSignals=Wheels.TireFrame.z,Wheels.Steering.WhlCmb,Wheels.TireFrame.Omega,Wheels.Steering.WhlAng
  Constant3 : Constant  Value=-ones(4,2).*.25*0
  Data Type Conversion{,5..7} (4 alike) : DataTypeConversion  OutDataTypeStr=double  SaturateOnIntegerOverflow=off  RndMeth=Floor
  Demux2 : Demux
  First Order Hold1 : FirstOrderHold  OutputAlgorithm=Fast (Minimize Error)  ErrorTolerance=.001
  First Order Hold9 : FirstOrderHold  InitialOutput=reshape(repmat(eye(3),1,1,4),[],1)  OutputAlgorithm=Fast (Minimize Error)  ErrorTolerance=.001
  For Each Subsystem : Subsystem  TreatAsAtomicUnit=on
  Integrator : Integrator  WrapState=on  ZeroCross=off
  Internal Tire Contact Plotter : vehdynlibviscommon/Internal Tire Contact Plotter  dispFig=on  numAxles=2  numWheelsPerAxle=2  wheelRad=.33  wheelWidth=.235  rayOrigins=rayOrigins
  Range Limiter{1..4} (4 alike) : Saturate  UpperLimit=1e3  LowerLimit=-1e3  ZeroCross=off
  Rate Transition1 : RateTransition  Integrity=off  Deterministic=off  OutPortSampleTime=.005
  Rate Transition2 : RateTransition  Integrity=off  Deterministic=off  OutPortSampleTime=.005
  Reshape : Reshape  OutputDimensionality=Column vector (2-D)
  Reshape1 : Reshape  OutputDimensionality=Column vector (2-D)
  Reshape2 : Reshape  OutputDimensionality=Row vector (2-D)
  Reshape3 : Reshape  OutputDimensionality=Row vector (2-D)
  Reshape4 : Reshape  OutputDimensionality=Row vector (2-D)
  Reshape5 : Reshape  OutputDimensionality=Customize  OutputDimensions=[3,3,4]
  Selector : Selector  NumberOfDimensions=2  InputPortWidth=3  IndexOptions=Select all,Index vector (dialog)  Indices=[1 3],3  OutputSizes=1,1
  Signal Specification{2..5} (4 alike) : SignalSpecification  Unit=m
  Simulation 3D Terrain Sensor : sim3dgroundtruthsensorlib/Simulation 3D Terrain Sensor  Priority=1  VehicleIdentifier=SimulinkVehicle1  vehTagList={'Scene Origin'}  sensorTag=Sim3dSensor1  sensorId=1  sensorName=Sim3dSensor1  vehTag=Scene Origin  tmountOffset=[0, 0, 0]  rmountOffset=[0,0,0,]  RayOrigins=rayOrigins  RayDirections=rayDirections  RayLengths=rayLengths  NumberOfWheels=4  VisualizeTraceLines=off  SampleTime=-1  aMode=2  ID=1
  Terminator : Terminator
  Unary Minus : UnaryMinus
  Vector Concatenate : Concatenate  NumInputs=4  Mode=Multidimensional array  ConcatenateDimension=3
  Vector Concatenate3 : Concatenate  Mode=Multidimensional array  ConcatenateDimension=2
  Vector Concatenate4 : Concatenate  NumInputs=3  Mode=Multidimensional array
  z : Outport
  DCM : Outport  Port=2
  wires:
  Data Type Conversion6/1 -> Vector Concatenate/3
  Range Limiter2/1 -> Data Type Conversion5/1
  Selector/1 -> First Order Hold1/1
  Signal Specification5/1 -> Bus Creator/4  "G_RR_z"
  Bus Selector1/3 -> Range Limiter3/1  "<Wheel3Positions>"
  Demux2/2 -> Signal Specification3/1
  Range Limiter3/1 -> Data Type Conversion6/1
  Data Type Conversion/1 -> Vector Concatenate/1
  Data Type Conversion5/1 -> Vector Concatenate/2
  Demux2/3 -> Signal Specification4/1
  Internal Tire Contact Plotter/1 -> Selector/1
  Internal Tire Contact Plotter/3 -> Terminator/1  "InContact"
  Vector Concatenate/1 -> Internal Tire Contact Plotter/1
  Data Type Conversion7/1 -> Vector Concatenate/4
  Bus Selector1/1 -> Range Limiter1/1  "<Wheel1Positions>"
  Range Limiter4/1 -> Data Type Conversion7/1
  Demux2/4 -> Signal Specification5/1
  Bus Creator/1 -> z/1  "z"
  Signal Specification2/1 -> Bus Creator/1  "G_FL_z"
  Bus Selector1/4 -> Range Limiter4/1  "<Wheel4Positions>"
  Signal Specification3/1 -> Bus Creator/2  "G_FR_z"
  Signal Specification4/1 -> Bus Creator/3  "G_RL_z"
  Bus Selector1/2 -> Range Limiter2/1  "<Wheel2Positions>"
  Demux2/1 -> Signal Specification2/1
  Simulation 3D Terrain Sensor/1 -> Bus Selector1/1
  Range Limiter1/1 -> Data Type Conversion/1
  Reshape5/1 -> DCM/1  "DCM"
  Internal Tire Contact Plotter/2 -> Reshape/1
  Bus Selector2/3 -> Reshape3/1  "<Omega>"
  Integrator/1 -> Unary Minus/1
  Bus Selector2/2 -> Reshape2/1  "<WhlCmb>"
  Vector Concatenate3/1 -> Rate Transition1/1
  For Each Subsystem/1(WheelDCM) -> Internal Tire Contact Plotter/3
  Reshape3/1 -> Integrator/1
  Vector Concatenate4/1 -> Rate Transition2/1
  Reshape4/1 -> Vector Concatenate4/3
  Rate Transition2/1 -> For Each Subsystem/1(phi,theta,psi)
  Reshape1/1 -> Vector Concatenate3/2
  VehFdbk/1 -> Bus Selector2/1
  Bus Selector2/1 -> Reshape1/1  "<z>"
  Bus Selector2/4 -> Reshape4/1  "<WhlAng>"
  Constant3/1 -> Vector Concatenate3/1
  Reshape2/1 -> Vector Concatenate4/1
  Unary Minus/1 -> Vector Concatenate4/2
  Rate Transition1/1 -> Internal Tire Contact Plotter/2
  First Order Hold9/1 -> Reshape5/1
  Reshape/1 -> First Order Hold9/1
  First Order Hold1/1 -> Demux2/1

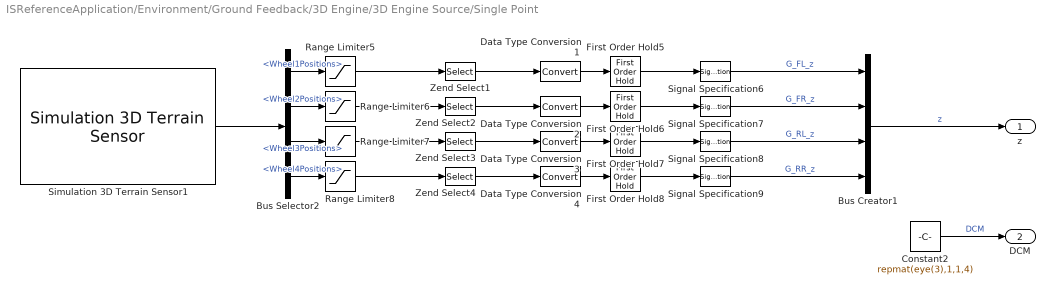
== system ISReferenceApplication/Environment/Ground Feedback/3D Engine/3D Engine Source/Single Point ==
  Bus Creator1 : BusCreator  Inputs=4
  Bus Selector2 : BusSelector  OutputSignals=Wheel1Positions,Wheel2Positions,Wheel3Positions,Wheel4Positions
  Constant2 : Constant  Value=repmat(eye(3),1,1,4)  SampleTime=-1
  Data Type Conversion{1..4} (4 alike) : DataTypeConversion  SaturateOnIntegerOverflow=off  RndMeth=Floor
  First Order Hold{5..8} (4 alike) : FirstOrderHold  ErrorTolerance=1
  Range Limiter{5..8} (4 alike) : Saturate  UpperLimit=1e3  LowerLimit=-1e3  ZeroCross=off
  Signal Specification{6..9} (4 alike) : SignalSpecification  Unit=m
  Simulation 3D Terrain Sensor1 : sim3dgroundtruthsensorlib/Simulation 3D Terrain Sensor  Priority=1  vehTagList={'Scene Origin';'SimulinkVehicle1'}  sensorTag=Sim3dSensor�  sensorId=1  sensorName=Sim3dSensor1  vehTag=SimulinkVehicle1  tmountOffset=[0, 0, 0]  rmountOffset=[0,0,0,]  RayOrigins=[0 0 1]  RayDirections=[0 0 -1]  RayLengths=20  NumberOfWheels=4  VisualizeTraceLines=off  SampleTime=-1  aMode=2  ID=1
  Zend Select{1..4} (4 alike) : Selector  NumberOfDimensions=2  InputPortWidth=3  IndexOptions=Select all,Index vector (dialog)  Indices=[1 3],3  OutputSizes=1,1
  z : Outport
  DCM : Outport  Port=2
  wires:
  Signal Specification6/1 -> Bus Creator1/1  "G_FL_z"
  Simulation 3D Terrain Sensor1/1 -> Bus Selector2/1
  Bus Selector2/4 -> Range Limiter8/1  "<Wheel4Positions>"
  Zend Select1/1 -> Data Type Conversion1/1
  Signal Specification7/1 -> Bus Creator1/2  "G_FR_z"
  Bus Selector2/2 -> Range Limiter6/1  "<Wheel2Positions>"
  Data Type Conversion3/1 -> First Order Hold7/1
  Data Type Conversion4/1 -> First Order Hold8/1
  Zend Select3/1 -> Data Type Conversion3/1
  First Order Hold6/1 -> Signal Specification7/1
  Zend Select2/1 -> Data Type Conversion2/1
  Data Type Conversion2/1 -> First Order Hold6/1
  Range Limiter6/1 -> Zend Select2/1
  Data Type Conversion1/1 -> First Order Hold5/1
  First Order Hold7/1 -> Signal Specification8/1
  Zend Select4/1 -> Data Type Conversion4/1
  Range Limiter8/1 -> Zend Select4/1
  Bus Selector2/1 -> Range Limiter5/1  "<Wheel1Positions>"
  First Order Hold8/1 -> Signal Specification9/1
  Bus Selector2/3 -> Range Limiter7/1  "<Wheel3Positions>"
  Range Limiter7/1 -> Zend Select3/1
  First Order Hold5/1 -> Signal Specification6/1
  Range Limiter5/1 -> Zend Select1/1
  Signal Specification8/1 -> Bus Creator1/3  "G_RL_z"
  Signal Specification9/1 -> Bus Creator1/4  "G_RR_z"
  Bus Creator1/1 -> z/1  "z"
  Constant2/1 -> DCM/1  "DCM"

== system ISReferenceApplication/Visualization/3D Engine/3D Engine/Scale/PartConcatenation ==
  BodyX : Inport
  BodyY : Inport  Port=2
  BodyZ : Inport  Port=3
  WheelFrontLeftX : Inport  Port=4
  WheelFrontLeftY : Inport  Port=5
  WheelFrontLeftZ : Inport  Port=6
  WheelFrontRightX : Inport  Port=7
  WheelFrontRightY : Inport  Port=8
  WheelFrontRightZ : Inport  Port=9
  WheelRearLeftX : Inport  Port=10
  WheelRearLeftY : Inport  Port=11
  WheelRearLeftZ : Inport  Port=12
  WheelRearRightX : Inport  Port=13
  WheelRearRightY : Inport  Port=14
  WheelRearRightZ : Inport  Port=15
  AllParts : Concatenate  NumInputs=5  Mode=Multidimensional array
  Body : Concatenate  NumInputs=3  Mode=Multidimensional array  ConcatenateDimension=2
  WheelFrontLeft : Concatenate  NumInputs=3  Mode=Multidimensional array  ConcatenateDimension=2
  WheelFrontRight : Concatenate  NumInputs=3  Mode=Multidimensional array  ConcatenateDimension=2
  WheelRearLeft : Concatenate  NumInputs=3  Mode=Multidimensional array  ConcatenateDimension=2
  WheelRearRight : Concatenate  NumInputs=3  Mode=Multidimensional array  ConcatenateDimension=2
  ConcatOut : Outport  VectorParamsAs1DForOutWhenUnconnected=off
  wires:
  BodyX/1 -> Body/1
  BodyZ/1 -> Body/3
  WheelFrontLeftX/1 -> WheelFrontLeft/1
  WheelFrontLeftZ/1 -> WheelFrontLeft/3
  WheelFrontLeftY/1 -> WheelFrontLeft/2
  BodyY/1 -> Body/2
  WheelFrontLeft/1 -> AllParts/2
  WheelRearRightX/1 -> WheelRearRight/1
  Body/1 -> AllParts/1
  WheelRearLeft/1 -> AllParts/4
  WheelFrontRight/1 -> AllParts/3
  WheelRearRightZ/1 -> WheelRearRight/3
  WheelFrontRightY/1 -> WheelFrontRight/2
  WheelFrontRightX/1 -> WheelFrontRight/1
  WheelRearRightY/1 -> WheelRearRight/2
  WheelRearLeftZ/1 -> WheelRearLeft/3
  AllParts/1 -> ConcatOut/1
  WheelRearLeftY/1 -> WheelRearLeft/2
  WheelRearRight/1 -> AllParts/5
  WheelRearLeftX/1 -> WheelRearLeft/1
  WheelFrontRightZ/1 -> WheelFrontRight/3

== system ISReferenceApplication/Environment/Ground Feedback/3D Engine/3D Engine Source/Multiple Points/For Each Subsystem ==
  phi,theta,psi : Inport  Partition=on  PartitionDimension=2  PartitionWidth=1  PartitionOffset=0
  For Each : ForEach  DisableCoverage=on
  Rotation Angles to Direction Cosine Matrix1 : sharedtransform/Rotation Angles to Direction Cosine Matrix  rotationOrder=YXZ  aMode=2
  Selector5 : Selector  InputPortWidth=3  IndexOptions=Index vector (dialog)  Indices=[2 1 3]  OutputSizes=1
  WheelDCM : Outport  ConcatenationDimension=3
  wires:
  Selector5/1 -> Rotation Angles to Direction Cosine Matrix1/1
  Rotation Angles to Direction Cosine Matrix1/1 -> WheelDCM/1
  phi,theta,psi/1 -> Selector5/1

== stateflow chart ISReferenceApplication/Controllers/Transmission Controller/Transmission Controller/TCM/TCM Shift Controller ==
  settings: sampleTime=0.01
  state GearCmd [parallel]
    settings: executionOrder=1
    state Neutral
      en:
      GearCmd = 0;
    state G1
      en:
      GearCmd = 1;
    state G2
      en:
      GearCmd = 2;
      du:
      [SpdThr] = calc(2,pedal,speed);
    state G3
      en:
      GearCmd = 3;
      du:
      [SpdThr] = calc(3,pedal,speed);
    state G8
      en:
      GearCmd = 8;
    state G7
      en:
      GearCmd = 7;
    state G6
      en:
      GearCmd = 6;
    state G5
      en:GearCmd=5;
      du:[SpdThr]=calc(5,pedal,speed);
    state G4
      en:
      GearCmd = 4;
      du:
      [SpdThr] = calc(4,pedal,speed);
    (default) -> Neutral
    Neutral -> G1 : [~Neutral]
    G1 -> G2 [order 1] : Up
    G2 -> G3 [order 1] : Up
    G1 -> Neutral [order 2] : [Neutral]
    G2 -> G1 [order 2] : Down
    G3 -> G2 [order 2] : Down
    G3 -> G4 [order 1] : Up
    G4 -> G3 [order 2] : Down
    G7 -> G8 [order 1] : Up
    G5 -> G6 [order 1] : Up
    G6 -> G7 [order 1] : Up
    G4 -> G5 [order 1] : Up
    G5 -> G4 [order 2] : Down
    G6 -> G5 [order 2] : Down
    G7 -> G6 [order 2] : Down
    G8 -> G7 : Down
  state SelectionState [parallel]
    du:[up_th]=calc_up(GearCmd,pedal);
    du:[down_th]=calc_down(GearCmd,pedal);
    settings: executionOrder=2
    state SteadyState
      en:
      clutchControl = 0;
    state preDownShifting
    state preUpShifting
    state UpShifting
      en:
      GearCmd = GearCmd + 0.5;
    state DownShifting
      en:
      GearCmd = GearCmd - 0.5;
    (default) -> SteadyState
    SteadyState -> (junction 62) [order 1] : [speed < down_th && ...
        | GearCmd >1]
    SteadyState -> (junction 128) [order 2] : [speed > up_th &&...
        | GearCmd <= 5 && ...
        | floor(GearCmd) == GearCmd]
    (junction 62) -> preDownShifting
    (junction 128) -> preUpShifting
    (junction 168) -> SteadyState
    (junction 23) -> SteadyState
    (junction 161) -> SteadyState
    preDownShifting -> (junction 168) [order 2] : [speed >= down_th]
    preUpShifting -> (junction 161) [order 2] : [speed <= up_th]
    preUpShifting -> UpShifting [order 1] : after(0.5,sec)
        | [speed>up_th]
    preDownShifting -> DownShifting [order 1] : after(0.5, sec)
        | [speed < down_th - 2]
    DownShifting -> (junction 23) : {GearCmd.Down;}
    UpShifting -> (junction 23) : {GearCmd.Up;}
  state up_th = calc_up(gear,pedal) [function]
  state down_th = calc_down(gear,pedal) [function]
  state SpdThr = calc(gear,pedal,speed) [function]
  data: gear function_input double size=1; pedal function_input double size=1; up_th function_output; gear function_input double size=1; pedal function_input double size=1; down_th function_output; gear function_input double size=1; pedal function_input double size=1; SpdThr function_output; speed function_input double size=1; GearCmd output int8; speed input; pedal input; clutchControl local double; SpdThr local double; Neutral input; up_th local double; down_th local double
  events: Up local EITHER_EDGE_EVENT; Down local EITHER_EDGE_EVENT

== stateflow chart ISReferenceApplication/Controllers/Brake Pressure Control/Five-State ABS and TCS/TCSCtrlForEach/For Each Subsystem/ABSForEachWheel ==
  state TCSOff
    entry:
    PbOutput = 0;
    Flag = 0;
    during:
    PbOutput = 0;
  state TCSRelease
    entry:
    PbOutput = v4;
  state Normal
    entry:
    PbOutput = 0;
    Flag = 0;
    during:
    PbOutput = 0;
  state TCSOn
    state Phase1
      entry:
      PbOutput = v1;
      Flag = 1;
    state Phase5
      entry:
      PbOutput = v5;
      Flag = 5;
    state Phase2
      entry:
      PbOutput = 0;
      Flag = 2;
    state Phase4
      entry:
      PbOutput = 0;
      Flag = 4;
    state Phase3
      entry:
      PbOutput = v4;
      Flag = 3;
    (default) -> Phase1
    Phase5 -> Phase1 : [e2 > a2]
    Phase1 -> Phase2 : [e2 <= b]
    Phase4 -> Phase5 : [e2 >= a1]
    Phase2 -> Phase3 : [e2 <= A]
    Phase3 -> Phase4 : [e2 > A]
  (default) -> TCSOff
  TCSRelease -> TCSOff : [Pb <= 0 || AccelFdbk <= 0.2]
  Normal -> TCSOff [order 2] : [AccelFdbk <= 0]
  TCSOn -> TCSRelease : [ AccelFdbk <= 0.2]
  TCSOff -> Normal : [AccelFdbk > 0 && e2 > a2 && Enb > 0.3]
  Normal -> TCSOn [order 1] : [e1 > 0]
  data: e1 input; e2 input; PbOutput output; Flag output; b parameter; v1 parameter; v4 parameter; v5 parameter; A parameter; a2 parameter; a1 parameter; AccelFdbk input; Enb input; Pb input

== matlab function ISReferenceApplication/Environment/MATLAB Function ==
  data: FLx input; FLy input; FRx input; FRy input; RLx input; RLy input; RRx input; RRy input; G_FL_z output; G_FR_z output; G_RL_z output; G_RR_z output
function [G_FL_z,G_FR_z,G_RL_z,G_RR_z] = roadloader(FLx,FLy,FRx,FRy,RLx,RLy,RRx,RRy)
    
    dir_name = "scenario/test_manhole/";


    %% Scenario csv path
    scenariopath = dir_name + "scenario_1_divp_Veh_NissanXtrail_1.csv";
    %% Pcdmap Path
    pcdmappath = dir_name + "map_gt.ply";

    G_FL_z = [0.0];
    G_FR_z = [0.0];
    G_RL_z = [0.0];
    G_RR_z = [0.0];

    FL = double([FLx, FLy]);
    FR = double([FRx, FRy]);
    RL = double([RLx, RLy]);
    RR = double([RRx, RRy]);

    coder.extrinsic('F_RoadLoader');
    [zfl,zfr,zrl,zrr] = F_RoadLoader(FL,FR,RL,RR,pcdmappath,scenariopath);

    G_FL_z = [double(zfl)];
    G_FR_z = [double(zfr)];
    G_RL_z = [double(zrl)];
    G_RR_z = [double(zrr)];
end
